simulink model "motion_sim"  (R2022a)
settings: Solver=FixedStepAuto  StartTime=0.0  StopTime=10.0  FixedStep=dof2_sim.dt  RelTol=1e-3
undefined symbols (not defined in the file): Iz, linear_actuator_force_torque_force_ratio, platform_mass
settings Model: Creator=mahdibabayi  LastModifiedBy=mahdibabayi

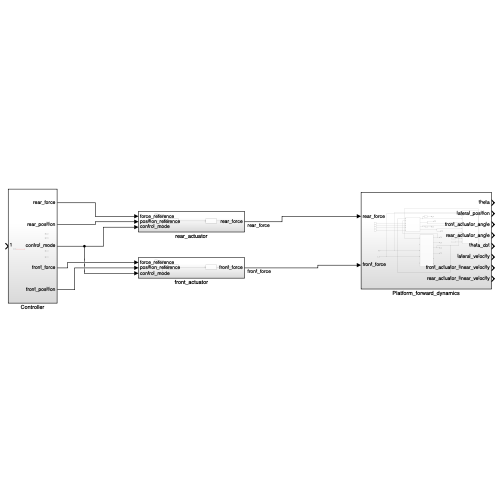
[thumbnail: Simulink's stored preview of the top-level diagram]
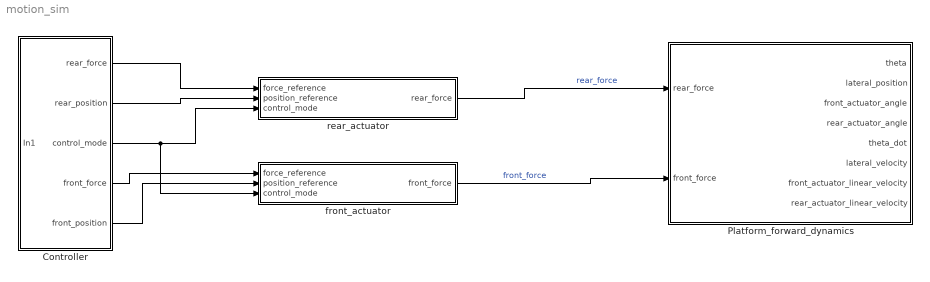
== system motion_sim ==
  Controller : Subsystem
  Platform_forward_dynamics : Subsystem
  front_actuator : Subsystem
  rear_actuator : Subsystem
  wires:
  rear_actuator/1(rear_force) -> Platform_forward_dynamics/1(rear_force)  "rear_force"
  front_actuator/1(front_force) -> Platform_forward_dynamics/2(front_force)  "front_force"
  Controller/1(rear_force) -> rear_actuator/1(force_reference)
  Controller/2(rear_position) -> rear_actuator/2(position_reference)
  Controller/4(front_force) -> front_actuator/1(force_reference)
  Controller/5(front_position) -> front_actuator/2(position_reference)
  Controller/3(control_mode) -> front_actuator/3(control_mode), rear_actuator/3(control_mode)

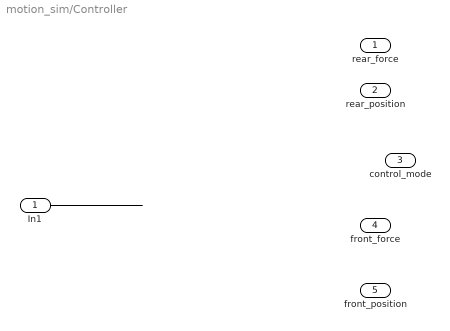
== system motion_sim/Controller ==
  In1 : Inport
  rear_force : Outport
  rear_position : Outport  Port=2
  control_mode : Outport  Port=3
  front_force : Outport  Port=4
  front_position : Outport  Port=5
  wires:
  In1/1 -> ?

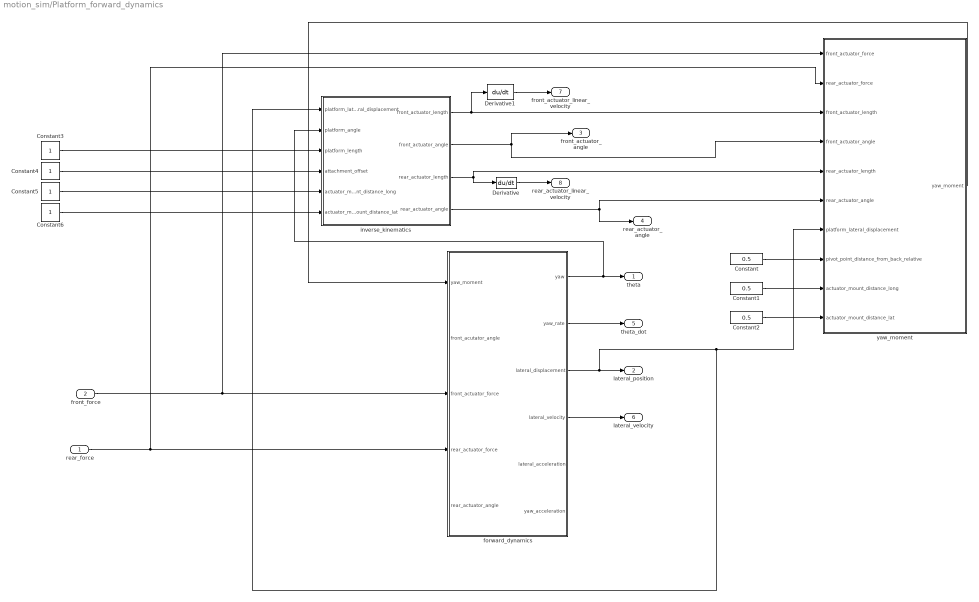
== system motion_sim/Platform_forward_dynamics ==
  rear_force : Inport
  front_force : Inport  Port=2
  Constant : Constant  Value=0.5
  Constant1 : Constant  Value=0.5
  Constant2 : Constant  Value=0.5
  Constant{3..6} (4 alike) : Constant
  Derivative : Derivative
  Derivative1 : Derivative
  forward_dynamics : Subsystem
  inverse_kinematics : MATLAB Function  TreatAsAtomicUnit=on
  yaw_moment : MATLAB Function  TreatAsAtomicUnit=on
  theta : Outport
  lateral_position : Outport  Port=2
  front_actuator_angle : Outport  Port=3
  rear_actuator_angle : Outport  Port=4
  theta_dot : Outport  Port=5
  lateral_velocity : Outport  Port=6
  front_actuator_linear_velocity : Outport  Port=7
  rear_actuator_linear_velocity : Outport  Port=8
  wires:
  inverse_kinematics/4(rear_actuator_angle) -> rear_actuator_angle/1, yaw_moment/6(rear_actuator_angle)
  inverse_kinematics/3(rear_actuator_length) -> Derivative/1, yaw_moment/5(rear_actuator_length)
  inverse_kinematics/1(front_actuator_length) -> Derivative1/1, yaw_moment/3(front_actuator_length)
  Derivative1/1 -> front_actuator_linear_velocity/1
  Derivative/1 -> rear_actuator_linear_velocity/1
  inverse_kinematics/2(front_actuator_angle) -> front_actuator_angle/1, yaw_moment/4(front_actuator_angle)
  yaw_moment/1(yaw_moment) -> forward_dynamics/1(yaw_moment)
  rear_force/1 -> yaw_moment/2(rear_actuator_force), forward_dynamics/4(rear_actuator_force)
  front_force/1 -> forward_dynamics/3(front_actuator_force), yaw_moment/1(front_actuator_force)
  forward_dynamics/1(yaw) -> inverse_kinematics/2(platform_angle), theta/1
  forward_dynamics/2(yaw_rate) -> theta_dot/1
  forward_dynamics/3(lateral_displacement) -> inverse_kinematics/1(platform_lateral_displacement), yaw_moment/7(platform_lateral_displacement), lateral_position/1
  forward_dynamics/4(lateral_velocity) -> lateral_velocity/1
  Constant/1 -> yaw_moment/8(pivot_point_distance_from_back_relative)
  Constant1/1 -> yaw_moment/9(actuator_mount_distance_long)
  Constant2/1 -> yaw_moment/10(actuator_mount_distance_lat)
  Constant3/1 -> inverse_kinematics/3(platform_length)
  Constant4/1 -> inverse_kinematics/4(attachment_offset)
  Constant5/1 -> inverse_kinematics/5(actuator_mount_distance_long)
  Constant6/1 -> inverse_kinematics/6(actuator_mount_distance_lat)

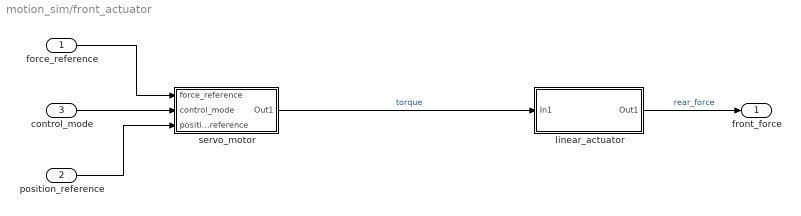
== system motion_sim/front_actuator ==
  force_reference : Inport
  position_reference : Inport  Port=2
  control_mode : Inport  Port=3
  linear_actuator : Subsystem
  servo_motor : Subsystem
  front_force : Outport
  wires:
  servo_motor/1(Out1) -> linear_actuator/1(In1)  "torque"
  control_mode/1 -> servo_motor/2(control_mode)
  force_reference/1 -> servo_motor/1(force_reference)
  position_reference/1 -> servo_motor/3(position_reference)
  linear_actuator/1(Out1) -> front_force/1  "rear_force"

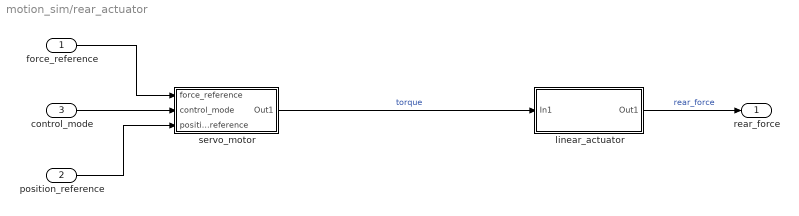
== system motion_sim/rear_actuator ==
  force_reference : Inport
  position_reference : Inport  Port=2
  control_mode : Inport  Port=3
  linear_actuator : Subsystem
  servo_motor : Subsystem
  rear_force : Outport
  wires:
  linear_actuator/1(Out1) -> rear_force/1  "rear_force"
  position_reference/1 -> servo_motor/3(position_reference)
  force_reference/1 -> servo_motor/1(force_reference)
  control_mode/1 -> servo_motor/2(control_mode)
  servo_motor/1(Out1) -> linear_actuator/1(In1)  "torque"

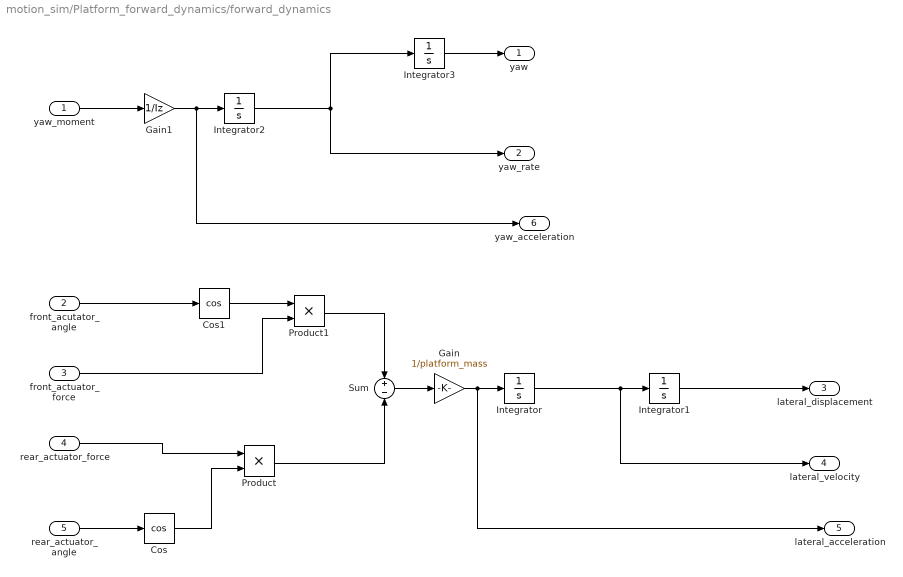
== system motion_sim/Platform_forward_dynamics/forward_dynamics ==
  yaw_moment : Inport
  front_acutator_angle : Inport  Port=2
  front_actuator_force : Inport  Port=3
  rear_actuator_force : Inport  Port=4
  rear_actuator_angle : Inport  Port=5
  Cos : Trigonometry  Operator=cos
  Cos1 : Trigonometry  Operator=cos
  Gain : Gain  Gain=1/platform_mass
  Gain1 : Gain  Gain=1/Iz
  Integrator{,1..3} (4 alike) : Integrator
  Product : Product
  Product1 : Product
  Sum : Sum  Inputs=+-
  yaw : Outport
  yaw_rate : Outport  Port=2
  lateral_displacement : Outport  Port=3
  lateral_velocity : Outport  Port=4
  lateral_acceleration : Outport  Port=5
  yaw_acceleration : Outport  Port=6
  wires:
  Integrator3/1 -> yaw/1
  rear_actuator_angle/1 -> Cos/1
  yaw_moment/1 -> Gain1/1
  front_acutator_angle/1 -> Cos1/1
  Cos1/1 -> Product1/1
  front_actuator_force/1 -> Product1/2
  rear_actuator_force/1 -> Product/1
  Cos/1 -> Product/2
  Sum/1 -> Gain/1
  Product/1 -> Sum/2
  Integrator1/1 -> lateral_displacement/1
  Gain/1 -> lateral_acceleration/1, Integrator/1
  Integrator/1 -> lateral_velocity/1, Integrator1/1
  Integrator2/1 -> yaw_rate/1, Integrator3/1
  Product1/1 -> Sum/1
  Gain1/1 -> yaw_acceleration/1, Integrator2/1

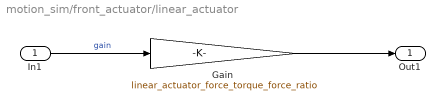
== system motion_sim/front_actuator/linear_actuator ==
  In1 : Inport
  Gain : Gain  Gain=linear_actuator_force_torque_force_ratio
  Out1 : Outport
  wires:
  Gain/1 -> Out1/1
  In1/1 -> Gain/1  "gain"

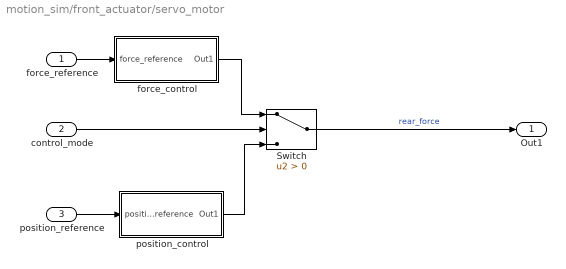
== system motion_sim/front_actuator/servo_motor ==
  force_reference : Inport
  control_mode : Inport  Port=2
  position_reference : Inport  Port=3
  Switch : Switch  Criteria=u2 > Threshold  SaturateOnIntegerOverflow=off  InputSameDT=off
  force_control : Subsystem
  position_control : Subsystem
  Out1 : Outport
  wires:
  Switch/1 -> Out1/1  "rear_force"
  control_mode/1 -> Switch/2
  position_reference/1 -> position_control/1(position_reference)
  force_reference/1 -> force_control/1(force_reference)
  force_control/1(Out1) -> Switch/1
  position_control/1(Out1) -> Switch/3

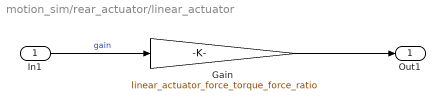
== system motion_sim/rear_actuator/linear_actuator ==
  In1 : Inport
  Gain : Gain  Gain=linear_actuator_force_torque_force_ratio
  Out1 : Outport
  wires:
  In1/1 -> Gain/1  "gain"
  Gain/1 -> Out1/1

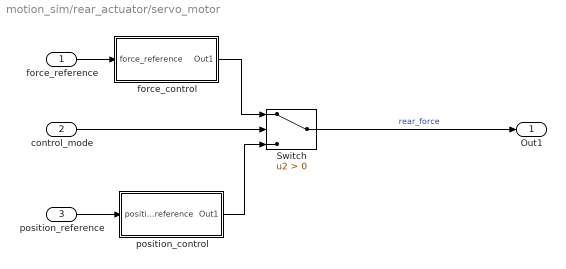
== system motion_sim/rear_actuator/servo_motor ==
  force_reference : Inport
  control_mode : Inport  Port=2
  position_reference : Inport  Port=3
  Switch : Switch  Criteria=u2 > Threshold  SaturateOnIntegerOverflow=off  InputSameDT=off
  force_control : Subsystem
  position_control : Subsystem
  Out1 : Outport
  wires:
  position_control/1(Out1) -> Switch/3
  force_control/1(Out1) -> Switch/1
  force_reference/1 -> force_control/1(force_reference)
  position_reference/1 -> position_control/1(position_reference)
  control_mode/1 -> Switch/2
  Switch/1 -> Out1/1  "rear_force"

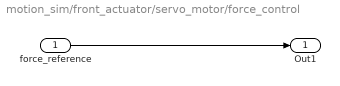
== system motion_sim/front_actuator/servo_motor/force_control ==
  force_reference : Inport
  Out1 : Outport
  wires:
  force_reference/1 -> Out1/1

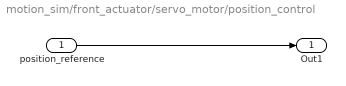
== system motion_sim/front_actuator/servo_motor/position_control ==
  position_reference : Inport
  Out1 : Outport
  wires:
  position_reference/1 -> Out1/1

== system motion_sim/rear_actuator/servo_motor/force_control ==
  force_reference : Inport
  Out1 : Outport
  wires:
  force_reference/1 -> Out1/1

== system motion_sim/rear_actuator/servo_motor/position_control ==
  position_reference : Inport
  Out1 : Outport
  wires:
  position_reference/1 -> Out1/1

== matlab function motion_sim/Platform_forward_dynamics/inverse_kinematics ==
  data: platform_lateral_displacement input; front_actuator_length output; platform_angle input; platform_length input; attachment_offset input; actuator_mount_distance_long input; actuator_mount_distance_lat input; front_actuator_angle output; rear_actuator_length output; rear_actuator_angle output
function [front_actuator_length,front_actuator_angle,rear_actuator_length, rear_actuator_angle] = fcn(...
                          platform_lateral_displacement,...
                          platform_angle,...
                          platform_length,...
                          attachment_offset,...
                          actuator_mount_distance_long,...
                          actuator_mount_distance_lat)
pivot_point_position = [actuator_mount_distance_long;actuator_mount_distance_lat + platform_lateral_displacement];
rear_actuator_mount_point = [0;0];
front_actuator_mount_point = [actuator_mount_distance_long;actuator_mount_distance_lat];
platform_rotation_matrix = [cos(platform_angle), -sin(platform_angle);...
                                            sin(platform_angle), cos(platform_angle)]; 
rear_actuator_end_point = pivot_point_position + platform_rotation_matrix*[-platform_length/2;attachment_offset];
front_actuator_end_point = pivot_point_position + platform_rotation_matrix * [platform_length/2;-attachment_offset];
front_actuator_vector = front_actuator_end_point - front_actuator_mount_point;
rear_actuator_vector = rear_actuator_end_point - rear_actuator_mount_point;
front_actuator_length = norm(front_actuator_vector);
rear_actuator_length = norm(rear_actuator_vector);
front_actuator_angle = atan2(-front_actuator_vector(2), -front_actuator_vector(1));
rear_actuator_angle = atan2(rear_actuator_vector(2) , rear_actuator_vector(1));
end

== matlab function motion_sim/Platform_forward_dynamics/yaw_moment ==
  data: front_actuator_force input; yaw_moment output; rear_actuator_force input; front_actuator_length input; front_actuator_angle input; rear_actuator_length input; rear_actuator_angle input; platform_lateral_displacement input; pivot_point_distance_from_back_relative input; actuator_mount_distance_long input; actuator_mount_distance_lat input
function yaw_moment = fcn(front_actuator_force,...
                          rear_actuator_force, ...
                          front_actuator_length, ...
                          front_actuator_angle,...
                          rear_actuator_length, ...
                          rear_actuator_angle,...
                          platform_lateral_displacement,...
                          pivot_point_distance_from_back_relative, ... 0 is in the back, 1 is in the front
                          actuator_mount_distance_long, ...
                          actuator_mount_distance_lat)
% returns yaw moment around pivot point
% assumes the hinge is mounted on the centre of mass
% assumes pivot point is half way between the actuator mount points
% using 3d vector to be able to use cross product for moment
com_position = [pivot_point_distance_from_back_relative*actuator_mount_distance_long;...
    actuator_mount_distance_lat/2 + platform_lateral_displacement;0 ];

rear_actuator_mount = [0;0;0];
rear_actuator_end_point = rear_actuator_length*[sin(rear_actuator_angle);cos(rear_actuato_angle);0];

front_actuator_mount = [actuator_mount_distance_long;actuator_mount_distance_lat;0];
front_actuator_end_point = front_actuator_mount - (front_actuator_length*[...
    sin(front_actuator_angle);cos(front_actuator_angle);0]);

rear_actuator_force_vector = ((rear_actuator_end_point - rear_actuator_mount)/rear_actuator_length) * rear_actuator_force;
front_actuator_force_vector = ((front_actuator_end_point - front_actuator_mount)/front_actuator_length)*front_actuator_force;
yaw_moment = cross(front_actuator_end_point - com_position , front_actuator_force_vector)+...
                        cross(rear_actuator_end_point - com_position, rear_actuator_force_vector);
yaw_moment = yaw_moment(3);

end
